simulink library "functionBezier_forward"  (R2024a)
settings: Solver=VariableStepAuto  StartTime=0.0  StopTime=10.0  RelTol=1e-3
settings Model: Creator=renre  LastModifiedBy=renre

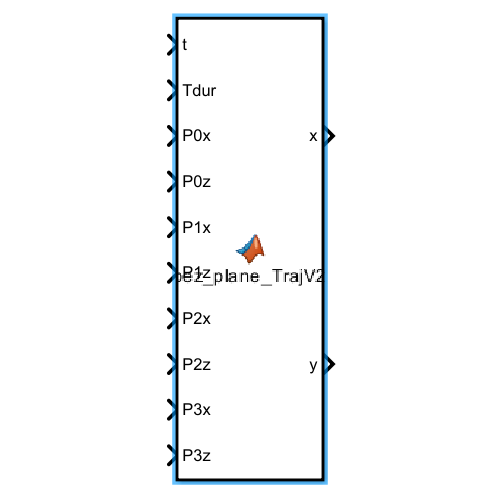
[thumbnail: Simulink's stored preview of the top-level diagram]
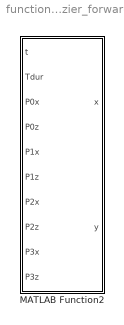
== system functionBezier_forward ==
  MATLAB Function2 : MATLAB Function  TreatAsAtomicUnit=on

== matlab function functionBezier_forward/MATLAB Function2 ==
  data: x output; t input; Tdur input; y output; P0x input; P0z input; P1x input; P1z input; P2x input; P2z input; P3x input; P3z input
function [x, y] = bez_plane_TrajV2(t,Tdur,P0x,P0z,P1x,P1z,P2x,P2z,P3x,P3z)
t_swing = Tdur/4;
t_support = Tdur*3/4;

P0 = [P0x, P0z];
P1 = [P1x, P1z];
P2 = [P2x, P2z];
P3 = [P3x, P3z];
P_ini = (P0 + P3)/2;

if Tdur == 0
    x = P_ini(1);
    y = P_ini(2);

elseif t<=t_support/2
    x = P_ini(1)-1*((P0(1)-P3(1))/t_support*(t));
    y = P_ini(2);

elseif t<=t_support/2+t_swing
    t_ef = (t-t_support/2);
    Sw = P0*((1-(t_ef/t_swing))^3) + 3*P1*(t_ef/t_swing)*((1-(t_ef/t_swing))^2) + 3*P2*((t_ef/t_swing)^2)*(1-(t_ef/t_swing)) + P3*((t_ef/t_swing)^3);
    
    x = -1*Sw(1);
    y = Sw(2);
else
    t_ef = (t-t_support/2-t_swing);
    x = -1*(P3(1)+(P0(1)-P3(1))/t_support*t_ef);
    y = P0(2);
end
end
